simulink model "CSE_StepResponse_ME_4203_Group1_2024_part2"  (R2023a)
settings: Solver=VariableStepAuto  StartTime=0.0  StopTime=10.0  RelTol=1e-3
values from neighbouring files (symbols this model uses):
  G_den = [M B K]    [CSE_StepResponse_ME_4203_Group1_2024_part1.m]    (also in CSE_StepResponse_ME_4203_Group1_2024_part2.m)
  G_num = [1]    [CSE_StepResponse_ME_4203_Group1_2024_part1.m]    (also in CSE_StepResponse_ME_4203_Group1_2024_part2.m)
settings Model: Creator=Willy  LastModifiedBy=Willy

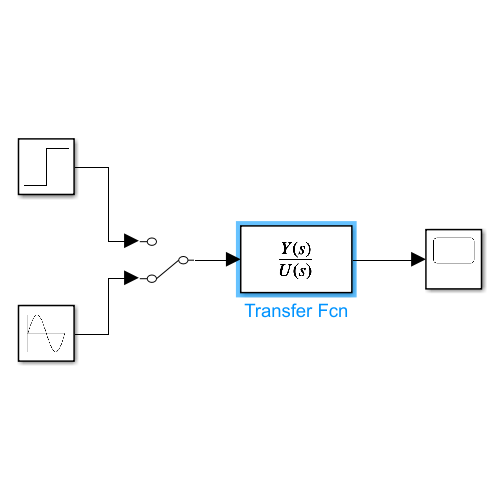
[thumbnail: Simulink's stored preview of the top-level diagram]
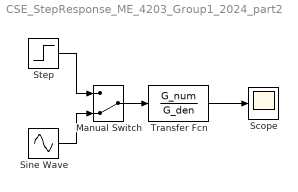
== system CSE_StepResponse_ME_4203_Group1_2024_part2 ==
  Manual Switch : ManualSwitch  CurrentSetting=0
  Scope : Scope
  Sine Wave : Sin  SampleTime=0
  Step : Step  SampleTime=0
  Transfer Fcn : TransferFcn  Numerator=G_num  Denominator=G_den
  wires:
  Manual Switch/1 -> Transfer Fcn/1
  Step/1 -> Manual Switch/1
  Sine Wave/1 -> Manual Switch/2
  Transfer Fcn/1 -> Scope/1
